simulink model "sampleModel1807"  (R2023a)
settings: Solver=VariableStepAuto  StartTime=0.0  StopTime=10.0  RelTol=1e-3
libraries: hdlsllib x4, simulink x2
settings Model: Creator=user1  LastModifiedBy=user1

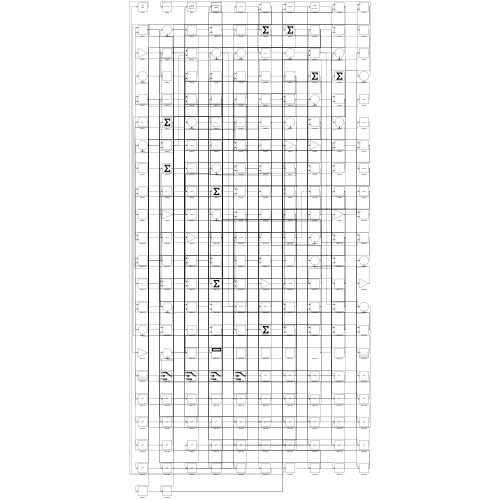
[thumbnail: Simulink's stored preview of the top-level diagram]
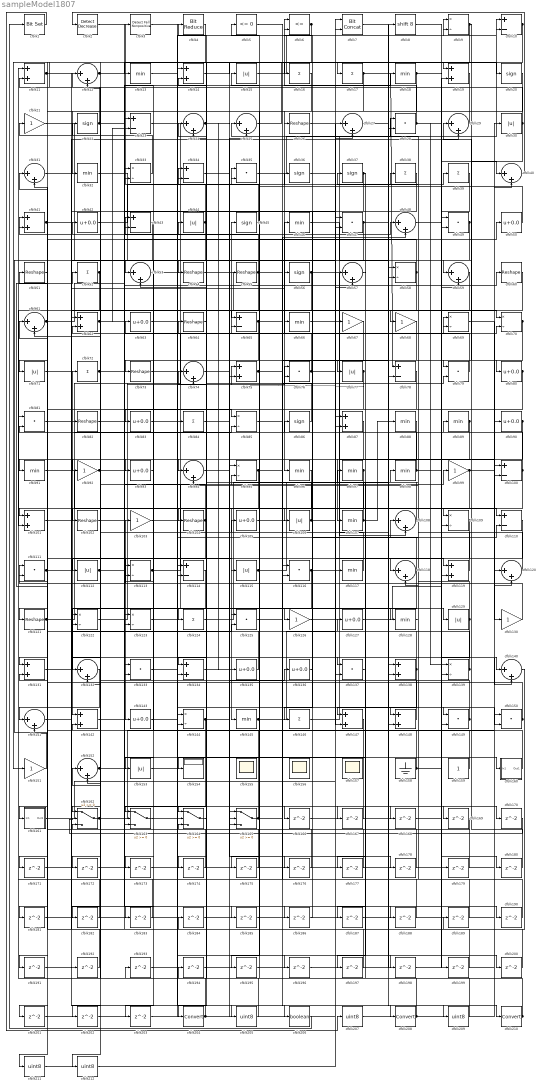
== system sampleModel1807 ==
  cfblk1 : simulink/Logic and Bit Operations/Bit Set  iBit=0
      settings: LibrarySourceBlock=|
      | hdlsllib/Logic and Bit
      | Operations/Bit Set
  cfblk{10,23,34,43,65,78,100,110,114} (9 alike) : Sum  Inputs=+-
  cfblk{11,14,19,41,62,75,87,101,119,131,134,138,142,147..148} (15 alike) : Sum
  cfblk{26,51,54..55,60,64,73,82,102,104,121} (11 alike) : Reshape
  cfblk{21,67..68,92,99,103,126,130,151} (9 alike) : Gain
  cfblk{42,50,63,80,83,90,93,105,127,135..136,143} (12 alike) : Bias  Bias=0.0  SaturateOnIntegerOverflow=off
  cfblk{15,30,44,71,77,106,112,115,129,153} (10 alike) : Abs  SaturateOnIntegerOverflow=off
  cfblk{13,18,32,46,66,88..89,91,96..98,107,117,128,145} (15 alike) : MinMax
  cfblk{12,24..25,27,29,31,40,48,53,57,59,61,74,94,108,118,120,132,140..141,152} (21 alike) : Sum  Inputs=|++
  cfblk{9,33,58,69..70,85,95,109,113,122..123,139,144} (13 alike) : Product  Inputs=*/  RndMeth=Zero  SaturateOnIntegerOverflow=on
  cfblk{28,35,47,49,76,79,81,111,116,125,133,137,149..150} (14 alike) : DotProduct  OutDataTypeStr=Inherit: Inherit via internal rule
  cfblk{16..17,38..39,52,72,84,124,146} (9 alike) : Sum  Inputs=+
  cfblk154 : Display
  cfblk155 : Scope
      settings: Floating=on
  cfblk156 : Scope
      settings: Floating=on
  cfblk157 : Scope
      settings: Floating=on
  cfblk158 : Ground
  cfblk159 : Constant  SampleTime=-1
  cfblk160 : Subsystem
      settings: LibrarySourceBlock=|
      | hdlsllib/Ports &
      | Subsystems/Subsystem
  cfblk161 : Subsystem
      settings: LibrarySourceBlock=|
      | hdlsllib/Ports &
      | Subsystems/Subsystem
  cfblk{162..165} (4 alike) : Switch  SaturateOnIntegerOverflow=off  InputSameDT=off
  cfblk{166..203} (38 alike) : Delay  SampleTime=1
  cfblk2 : simulink/Logic and Bit Operations/Detect Decrease  vinit=0.0  OutDataTypeStr=boolean
      settings: LibrarySourceBlock=|
      | hdlsllib/Logic and Bit
      | Operations/Detect
      | Decrease
  cfblk{20,22,36..37,45,56,86} (7 alike) : Signum
  cfblk204 : DataTypeConversion  SaturateOnIntegerOverflow=off  RndMeth=Floor
  cfblk{205,207,209,211..212} (5 alike) : DataTypeConversion  OutDataTypeStr=uint8  SaturateOnIntegerOverflow=off  RndMeth=Floor
  cfblk206 : DataTypeConversion  OutDataTypeStr=boolean  SaturateOnIntegerOverflow=off  RndMeth=Floor
  cfblk208 : DataTypeConversion  SaturateOnIntegerOverflow=off  RndMeth=Floor
  cfblk210 : DataTypeConversion  SaturateOnIntegerOverflow=off  RndMeth=Floor
  cfblk3 : hdlsllib/Logic and Bit Operations/Detect Fall Nonpositive  vinit=0  OutDataTypeStr=boolean
  cfblk4 : hdlsllib/Logic and Bit Operations/Bit Reduce  mode=AND
  cfblk5 : hdlsllib/Logic and Bit Operations/Compare To Zero  relop=<=  OutDataTypeStr=boolean
  cfblk6 : RelationalOperator  Operator=<=  OutDataTypeStr=boolean  InputSameDT=off
  cfblk7 : hdlsllib/Logic and Bit Operations/Bit Concat  numInputs=2
  cfblk8 : ArithShift  BitShiftNumber=8
  wires:
  cfblk18/1 -> cfblk96/1, cfblk140/1, cfblk101/1, cfblk195/1, cfblk211/1
  cfblk146/1 -> cfblk10/1
  cfblk129/1 -> cfblk111/1, cfblk139/2, cfblk94/2
  cfblk87/1 -> cfblk91/1
  cfblk147/1 -> cfblk52/1
  cfblk138/1 -> cfblk154/1, cfblk35/2
  cfblk80/1 -> cfblk94/1, cfblk174/1, cfblk175/1
  cfblk131/1 -> cfblk72/1
  cfblk151/1 -> cfblk53/1
  cfblk113/1 -> cfblk99/1, cfblk198/1
  cfblk110/1 -> cfblk143/1
  cfblk70/1 -> cfblk80/1, cfblk177/1
  cfblk56/1 -> cfblk108/2, cfblk202/1
  cfblk23/1 -> cfblk126/1
  cfblk25/1 -> cfblk19/1
  cfblk17/1 -> cfblk78/1, cfblk132/2
  cfblk40/1 -> cfblk2/1
  cfblk35/1 -> cfblk28/1
  cfblk122/1 -> cfblk76/1
  cfblk63/1 -> cfblk14/1
  cfblk45/1 -> cfblk3/1
  cfblk160/1(Out1) -> cfblk33/1
  cfblk130/1 -> cfblk103/1
  cfblk104/1 -> cfblk131/1, cfblk22/1
  cfblk128/1 -> cfblk98/1
  cfblk83/1 -> cfblk129/1
  cfblk133/1 -> cfblk144/2
  cfblk152/1 -> cfblk30/1, cfblk18/1
  cfblk109/1 -> cfblk118/1, cfblk163/2
  cfblk90/1 -> cfblk107/1, cfblk212/1
  cfblk105/1 -> cfblk110/1
  cfblk32/1 -> cfblk114/1
  cfblk68/1 -> cfblk73/1
  cfblk60/1 -> cfblk121/1
  cfblk69/1 -> cfblk100/1
  cfblk126/1 -> cfblk58/1
  cfblk33/1 -> cfblk21/1
  cfblk115/1 -> cfblk8/1, cfblk200/1
  cfblk7/1 -> cfblk210/1
  cfblk22/1 -> cfblk151/1, cfblk57/2, cfblk165/3
  cfblk117/1 -> cfblk12/1
  cfblk145/1 -> cfblk27/1, cfblk79/2
  cfblk164/1 -> cfblk44/1
  cfblk21/1 -> cfblk84/1
  cfblk142/1 -> cfblk95/2
  cfblk99/1 -> cfblk90/1, cfblk134/2
  cfblk95/1 -> cfblk164/1, cfblk148/1, cfblk35/1
  cfblk137/1 -> cfblk97/1
  cfblk5/1 -> cfblk208/1
  cfblk86/1 -> cfblk4/1
  cfblk124/1 -> cfblk57/1
  cfblk47/1 -> cfblk104/1, cfblk150/2
  cfblk111/1 -> cfblk45/1, cfblk115/1, cfblk137/2
  cfblk102/1 -> cfblk60/1
  cfblk19/1 -> cfblk32/1
  cfblk120/1 -> cfblk25/1
  cfblk57/1 -> cfblk147/1
  cfblk149/1 -> cfblk24/1, cfblk61/2, cfblk113/2
  cfblk24/1 -> cfblk70/1, cfblk135/1
  cfblk98/1 -> cfblk86/1, cfblk180/1
  cfblk46/1 -> cfblk138/1
  cfblk79/1 -> cfblk63/1
  cfblk135/1 -> cfblk33/2
  cfblk76/1 -> cfblk46/1, cfblk148/2
  cfblk12/1 -> cfblk123/1, cfblk16/1
  cfblk11/1 -> cfblk47/2, cfblk209/1
  cfblk55/1 -> cfblk13/1, cfblk41/2, cfblk101/2, cfblk92/1, cfblk137/1
  cfblk27/1 -> cfblk100/2
  cfblk127/1 -> cfblk49/1
  cfblk15/1 -> cfblk10/2
  cfblk31/1 -> cfblk65/1
  cfblk132/1 -> cfblk141/1
  cfblk9/1 -> cfblk59/1, cfblk152/2
  cfblk106/1 -> cfblk82/1, cfblk70/2
  cfblk61/1 -> cfblk48/1, cfblk55/1
  cfblk114/1 -> cfblk142/1
  cfblk2/1 -> cfblk109/1
  cfblk26/1 -> cfblk119/1
  cfblk103/1 -> cfblk149/1
  cfblk71/1 -> cfblk128/1
  cfblk82/1 -> cfblk27/2
  cfblk50/1 -> cfblk15/1
  cfblk10/1 -> cfblk17/1, cfblk124/1
  cfblk136/1 -> cfblk66/1
  cfblk41/1 -> cfblk140/2, cfblk188/1
  cfblk112/1 -> cfblk42/1, cfblk50/1
  cfblk62/1 -> cfblk85/1, cfblk23/2
  cfblk159/1 -> cfblk131/2
  cfblk67/1 -> cfblk123/2
  cfblk44/1 -> cfblk34/1, cfblk122/2, cfblk112/1, cfblk163/3
  cfblk20/1 -> cfblk54/1
  cfblk107/1 -> cfblk53/2, cfblk88/1
  cfblk39/1 -> cfblk49/2
  cfblk89/1 -> cfblk106/1, cfblk147/2
  cfblk38/1 -> cfblk146/1
  cfblk59/1 -> cfblk71/1
  cfblk13/1 -> cfblk9/1
  cfblk108/1 -> cfblk62/2, cfblk81/2
  cfblk52/1 -> cfblk132/1, cfblk141/2
  cfblk148/1 -> cfblk74/1
  cfblk121/1 -> cfblk85/2, cfblk125/2
  cfblk100/1 -> cfblk43/1, cfblk187/1
  cfblk66/1 -> cfblk130/1
  cfblk75/1 -> cfblk168/1, cfblk169/1
  cfblk163/1 -> cfblk110/2
  cfblk81/1 -> cfblk29/2
  cfblk6/1 -> cfblk161/1(In1), cfblk165/2
  cfblk162/1 -> cfblk67/1, cfblk56/1
  cfblk161/1(Out1) -> cfblk87/1
  cfblk28/1 -> cfblk40/1, cfblk6/2, cfblk139/1
  cfblk77/1 -> cfblk113/1, cfblk74/2
  cfblk14/1 -> cfblk20/1
  cfblk43/1 -> cfblk102/1
  cfblk119/1 -> cfblk37/1
  cfblk65/1 -> cfblk78/2, cfblk83/1
  cfblk92/1 -> cfblk38/1, cfblk69/2
  cfblk125/1 -> cfblk48/2
  cfblk30/1 -> cfblk11/2, cfblk79/1
  cfblk97/1 -> cfblk145/1, cfblk153/1
  cfblk116/1 -> cfblk162/1, cfblk39/1
  cfblk123/1 -> cfblk34/2
  cfblk158/1 -> cfblk105/1, cfblk59/2
  cfblk118/1 -> cfblk6/1, cfblk203/1
  cfblk49/1 -> cfblk93/1, cfblk182/1
  cfblk36/1 -> cfblk9/2
  cfblk42/1 -> cfblk36/1
  cfblk150/1 -> cfblk89/1, cfblk41/1
  cfblk53/1 -> cfblk125/1
  cfblk64/1 -> cfblk204/1
  cfblk72/1 -> cfblk160/1(In1), cfblk185/1
  cfblk37/1 -> cfblk133/2, cfblk77/1, cfblk75/2
  cfblk54/1 -> cfblk68/1
  cfblk144/1 -> cfblk136/1, cfblk173/1
  cfblk91/1 -> cfblk116/2
  cfblk143/1 -> cfblk75/1
  cfblk139/1 -> cfblk51/1, cfblk14/2
  cfblk84/1 -> cfblk165/1
  cfblk74/1 -> cfblk69/1
  cfblk29/1 -> cfblk26/1
  cfblk165/1 -> cfblk43/2, cfblk178/1
  cfblk58/1 -> cfblk163/1, cfblk134/1, cfblk31/2
  cfblk34/1 -> cfblk166/1
  cfblk166/1 -> cfblk19/2
  cfblk85/1 -> cfblk167/1
  cfblk167/1 -> cfblk122/1
  cfblk168/1 -> cfblk109/2
  cfblk169/1 -> cfblk162/3
  cfblk134/1 -> cfblk170/1
  cfblk170/1 -> cfblk162/2
  cfblk78/1 -> cfblk171/1
  cfblk171/1 -> cfblk23/1
  cfblk16/1 -> cfblk172/1
  cfblk172/1 -> cfblk40/2
  cfblk173/1 -> cfblk119/2
  cfblk174/1 -> cfblk144/1
  cfblk175/1 -> cfblk164/3
  cfblk94/1 -> cfblk176/1
  cfblk176/1 -> cfblk31/1
  cfblk177/1 -> cfblk65/2
  cfblk178/1 -> cfblk24/2
  cfblk48/1 -> cfblk179/1
  cfblk179/1 -> cfblk108/1
  cfblk180/1 -> cfblk29/1
  cfblk4/1 -> cfblk181/1
  cfblk181/1 -> cfblk114/2
  cfblk182/1 -> cfblk111/2
  cfblk93/1 -> cfblk183/1
  cfblk183/1 -> cfblk11/1
  cfblk184/1 -> cfblk58/2
  cfblk185/1 -> cfblk47/1
  cfblk141/1 -> cfblk186/1
  cfblk186/1 -> cfblk76/2
  cfblk187/1 -> cfblk150/1
  cfblk188/1 -> cfblk116/1
  cfblk140/1 -> cfblk189/1
  cfblk189/1 -> cfblk152/1
  cfblk73/1 -> cfblk190/1
  cfblk190/1 -> cfblk118/2
  cfblk96/1 -> cfblk191/1
  cfblk101/1 -> cfblk192/1
  cfblk192/1 -> cfblk61/1
  cfblk193/1 -> cfblk28/2
  cfblk194/1 -> cfblk149/2
  cfblk195/1 -> cfblk87/2
  cfblk153/1 -> cfblk196/1
  cfblk196/1 -> cfblk138/2
  cfblk88/1 -> cfblk197/1
  cfblk197/1 -> cfblk133/1
  cfblk198/1 -> cfblk120/2
  cfblk8/1 -> cfblk199/1
  cfblk199/1 -> cfblk62/1
  cfblk200/1 -> cfblk142/2
  cfblk51/1 -> cfblk201/1
  cfblk201/1 -> cfblk95/1
  cfblk202/1 -> cfblk164/2
  cfblk203/1 -> cfblk25/2
  cfblk204/1 -> cfblk81/1, cfblk117/1, cfblk12/2
  cfblk3/1 -> cfblk205/1
  cfblk205/1 -> cfblk64/1
  cfblk191/1 -> cfblk206/1
  cfblk206/1 -> cfblk1/1
  cfblk1/1 -> cfblk207/1
  cfblk207/1 -> cfblk120/1
  cfblk208/1 -> cfblk184/1, cfblk127/1
  cfblk209/1 -> cfblk5/1
  cfblk210/1 -> cfblk194/1, cfblk193/1
  cfblk211/1 -> cfblk7/1
  cfblk212/1 -> cfblk7/2

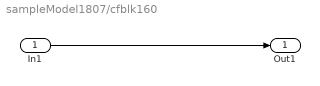
== system sampleModel1807/cfblk160 ==
  In1 : Inport
  Out1 : Outport
  wires:
  In1/1 -> Out1/1

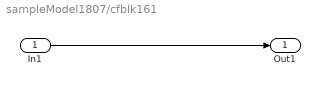
== system sampleModel1807/cfblk161 ==
  In1 : Inport
  Out1 : Outport
  wires:
  In1/1 -> Out1/1
